simulink model "lab05es01e1_errore_inseguimento"  (R2021b)
settings: Solver=VariableStepAuto  StartTime=0.0  StopTime=30.0  RelTol=1e-3
values from neighbouring files (symbols this model uses):
  Kc = Kr/(Kf*0.2)    [L_11_05_21_reti_anticipatrici.m]    (also in L_11_05_21_reti_anticipatrici_2.m; L_12_05_21_Esercizio_progetto_di_un_controllore.m = 1/(0.04*Kf1*Kf2); L_12_05_21_effetti_sul_comando.m = 4; L_12_05_21_reti_integro-derivative.m = 4)
  Kr = 1    [L_11_05_21_reti_anticipatrici.m]    (also in L_11_05_21_reti_anticipatrici_2.m; L_12_05_21_Esercizio_progetto_di_un_controllore.m; L_12_05_21_effetti_sul_comando.m; L_12_05_21_reti_integro-derivative.m)
libraries: cstblocks x1, simulink x1
settings Model: Creator=francescafornasier  LastModifiedBy=francescafornasier

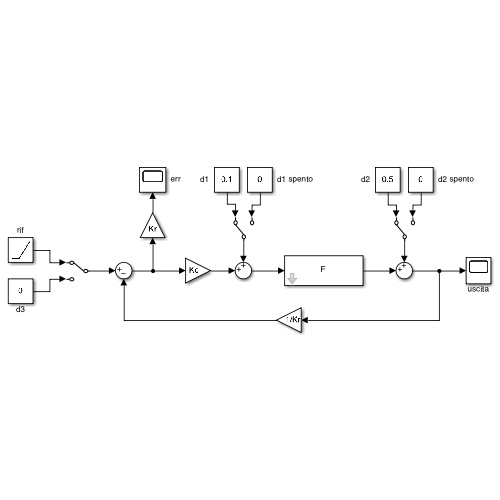
[thumbnail: Simulink's stored preview of the top-level diagram]
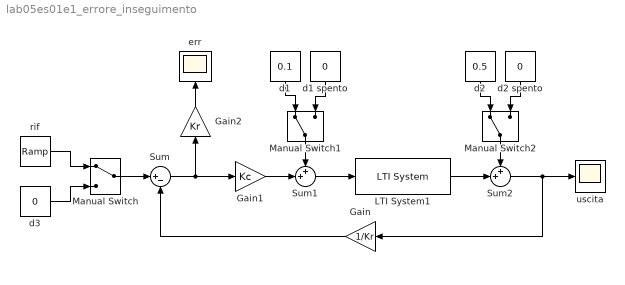
== system lab05es01e1_errore_inseguimento ==
  Gain : Gain  Gain=1/Kr
  Gain1 : Gain  Gain=Kc
  Gain2 : Gain  Gain=Kr
  LTI System1 : cstblocks/LTI System  sys=F  IC=[]
  Manual Switch : ManualSwitch
  Manual Switch1 : ManualSwitch
  Manual Switch2 : ManualSwitch
  Sum : Sum  Inputs=|+-
  Sum1 : Sum  Inputs=++|
  Sum2 : Sum  Inputs=++|
  d1 : Constant  Value=0.1
  d1 spento : Constant  Value=0
  d2 : Constant  Value=0.5
  d2 spento : Constant  Value=0
  d3 : Constant  Value=0
  err : Scope
  rif : simulink/Sources/Ramp  slope=1  start=0  InitialOutput=0
  uscita : Scope
  wires:
  Gain1/1 -> Sum1/2
  Gain/1 -> Sum/2
  Sum1/1 -> LTI System1/1
  LTI System1/1 -> Sum2/2
  Sum2/1 -> Gain/1, uscita/1
  Manual Switch/1 -> Sum/1
  rif/1 -> Manual Switch/1
  d3/1 -> Manual Switch/2
  Manual Switch1/1 -> Sum1/1
  Manual Switch2/1 -> Sum2/1
  d2/1 -> Manual Switch2/1
  d1/1 -> Manual Switch1/1
  d1 spento/1 -> Manual Switch1/2
  d2 spento/1 -> Manual Switch2/2
  Sum/1 -> Gain2/1, Gain1/1
  Gain2/1 -> err/1
